simulink model "SSmodel_LQG_regulator"  (Simulink 7.5)
settings: Solver=ode45  StartTime=0.0  StopTime=3  FixedStep=Ts  MaxStep=1e-2  RelTol=1e-3
values from neighbouring files (symbols this model uses):
  d_w = 0.00005    (= 5e-05)    [TSC160127ProvaMatlab.m]
  d_y = 0.00001    (= 1e-05)    [TSC160127ProvaMatlab.m]
  L = -LKalman    [TSC160127ProvaMatlab.m]
  Xl0 = [0.03;0]    [TSC160127ProvaMatlab.m]
undefined symbols (not defined in the file or in its folder): A, B, C, K
settings Model: Creator=lbiagiotti  LastModifiedBy=Biagio
settings DebuggingCC: SaveWithParameterizedLinksMsg=none  StrictBusMsg=Warning
settings HardwareCC: TargetHWDeviceType=32-bit Generic
settings GRTTargetCC: TargetFcnLib=ansi_tfl_tmw.mat

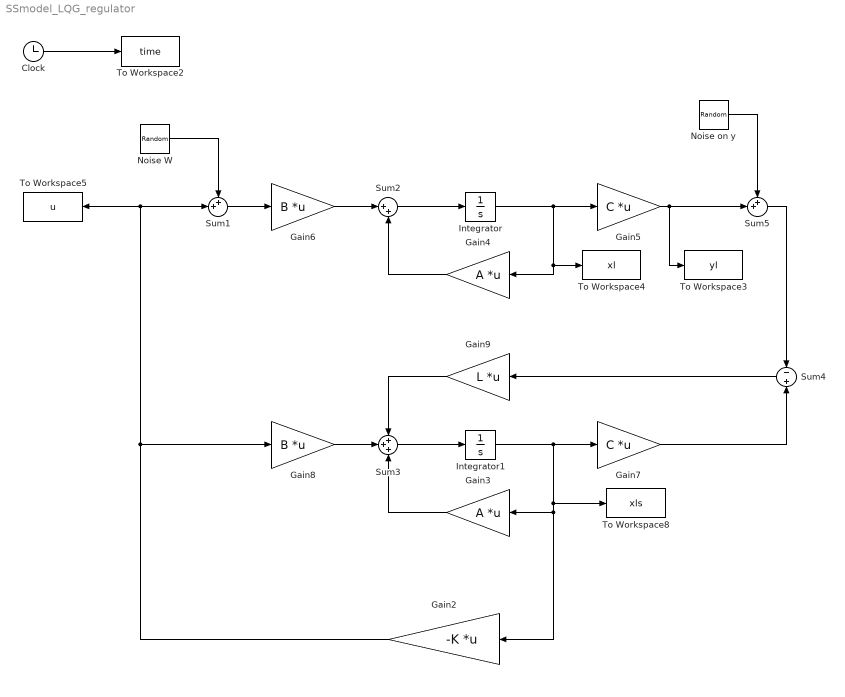
== system SSmodel_LQG_regulator ==
  Clock : Clock
      settings: Decimation=10
  Gain2 : Gain  Gain=-K  Multiplication=Matrix(K*u)  ParameterDataType=sfix(16)  ParameterScaling=2^0  OutDataType=sfix(16)  OutScaling=2^0
  Gain3 : Gain  Gain=A  Multiplication=Matrix(K*u)  ParameterDataType=sfix(16)  ParameterScaling=2^0  OutDataType=sfix(16)  OutScaling=2^0
  Gain4 : Gain  Gain=A  Multiplication=Matrix(K*u)  ParameterDataType=sfix(16)  ParameterScaling=2^0  OutDataType=sfix(16)  OutScaling=2^0
  Gain5 : Gain  Gain=C  Multiplication=Matrix(K*u)  ParameterDataType=sfix(16)  ParameterScaling=2^0  OutDataType=sfix(16)  OutScaling=2^0
  Gain6 : Gain  Gain=B  Multiplication=Matrix(K*u)  ParameterDataType=sfix(16)  ParameterScaling=2^0  OutDataType=sfix(16)  OutScaling=2^0
  Gain7 : Gain  Gain=C  Multiplication=Matrix(K*u)  ParameterDataType=sfix(16)  ParameterScaling=2^0  OutDataType=sfix(16)  OutScaling=2^0
  Gain8 : Gain  Gain=B  Multiplication=Matrix(K*u)  ParameterDataType=sfix(16)  ParameterScaling=2^0  OutDataType=sfix(16)  OutScaling=2^0
  Gain9 : Gain  Gain=L  Multiplication=Matrix(K*u)  ParameterDataType=sfix(16)  ParameterScaling=2^0  OutDataType=sfix(16)  OutScaling=2^0
  Integrator : Integrator  InitialCondition=Xl0
  Integrator1 : Integrator  InitialCondition=[0 0]'
  Noise W : RandomNumber  Variance=d_w  SampleTime=0
  Noise on y : RandomNumber  Variance=d_y  SampleTime=0
  Sum1 : Sum  Inputs=++|  OutDataType=fixdt(1, 16)  OutScaling=2^0
  Sum2 : Sum  Inputs=|++  OutDataType=sfix(16)  OutScaling=2^0
  Sum3 : Sum  Inputs=+++  OutDataType=sfix(16)  OutScaling=2^0
  Sum4 : Sum  Inputs=-+  OutDataType=sfix(16)  OutScaling=2^0
  Sum5 : Sum  Inputs=++|  OutDataType=fixdt(1, 16)  OutScaling=2^0
  To Workspace2 : ToWorkspace  VariableName=time  SampleTime=-1  SaveFormat=Array
  To Workspace3 : ToWorkspace  VariableName=yl  SampleTime=-1  SaveFormat=Array
  To Workspace4 : ToWorkspace  VariableName=xl  SampleTime=-1  SaveFormat=Array
  To Workspace5 : ToWorkspace  VariableName=u  SampleTime=-1  SaveFormat=Array
  To Workspace8 : ToWorkspace  VariableName=xls  SampleTime=-1  SaveFormat=Array
  wires:
  Gain6/1 -> Sum2/1
  Gain4/1 -> Sum2/2
  Sum2/1 -> Integrator/1
  Integrator/1 -> To Workspace4/1, Gain4/1, Gain5/1
  Clock/1 -> To Workspace2/1
  Gain2/1 -> Gain8/1, To Workspace5/1, Sum1/2
  Sum3/1 -> Integrator1/1
  Integrator1/1 -> Gain7/1, To Workspace8/1, Gain3/1, Gain2/1
  Gain7/1 -> Sum4/2
  Gain9/1 -> Sum3/1
  Gain8/1 -> Sum3/2
  Gain3/1 -> Sum3/3
  Sum4/1 -> Gain9/1
  Noise W/1 -> Sum1/1
  Sum1/1 -> Gain6/1
  Noise on y/1 -> Sum5/1
  Gain5/1 -> To Workspace3/1, Sum5/2
  Sum5/1 -> Sum4/1
